simulink model "da2863_HW4_Simulink"  (R2023b)
settings: Solver=ode4  StartTime=0.0  StopTime=60  FixedStep=0.001  RelTol=1e-3
settings Model: Creator=Dhiya  LastModifiedBy=Dhiya

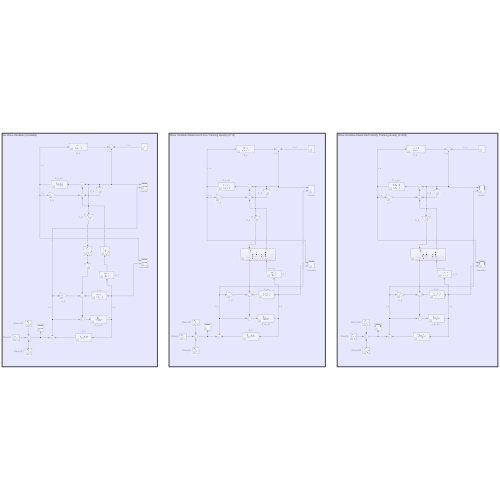
[thumbnail: Simulink's stored preview of the top-level diagram]
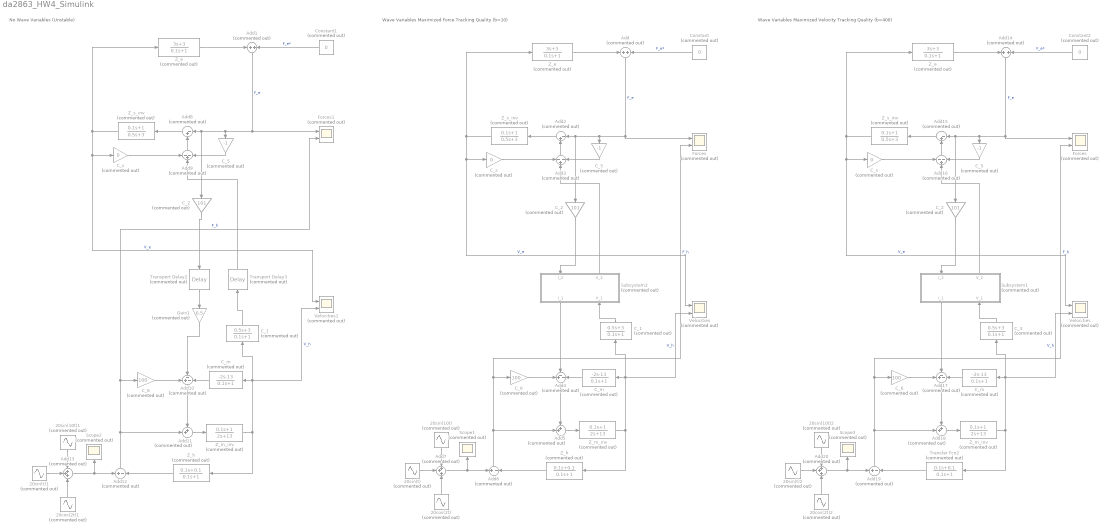
== system da2863_HW4_Simulink ==
  note: Wave Variables Maximized Velocity Tracking Quality (b=400)
  note: Wave Variables Maximized Force Tracking Quality (b=10)
  note: No Wave Variables (Unstable)
  20cos(2t) : Sin  Commented=on  Amplitude=20  Frequency=2  Phase=pi/2  SampleTime=0
  20cos(2t)1 : Sin  Commented=on  Amplitude=20  Frequency=2  Phase=pi/2  SampleTime=0
  20cos(2t)2 : Sin  Commented=on  Amplitude=20  Frequency=2  Phase=pi/2  SampleTime=0
  20sin(10t) : Sin  Commented=on  Amplitude=20  Frequency=10  SampleTime=0
  20sin(10t)1 : Sin  Commented=on  Amplitude=20  Frequency=10  SampleTime=0
  20sin(10t)2 : Sin  Commented=on  Amplitude=20  Frequency=10  SampleTime=0
  20sin(t) : Sin  Commented=on  Amplitude=20  SampleTime=0
  20sin(t)1 : Sin  Commented=on  Amplitude=20  SampleTime=0
  20sin(t)2 : Sin  Commented=on  Amplitude=20  SampleTime=0
  Add : Sum  Commented=on  Inputs=+|+
  Add1 : Sum  Commented=on  Inputs=+|+
  Add10 : Sum  Commented=on  Inputs=+--
  Add11 : Sum  Commented=on  Inputs=++|
  Add12 : Sum  Commented=on  Inputs=+|-
  Add13 : Sum  Commented=on  Inputs=+++
  Add14 : Sum  Commented=on  Inputs=+|+
  Add15 : Sum  Commented=on  Inputs=|-+
  Add16 : Sum  Commented=on  Inputs=-+-
  Add17 : Sum  Commented=on  Inputs=+--
  Add18 : Sum  Commented=on  Inputs=++|
  Add19 : Sum  Commented=on  Inputs=+|-
  Add2 : Sum  Commented=on  Inputs=|-+
  Add20 : Sum  Commented=on  Inputs=+++
  Add3 : Sum  Commented=on  Inputs=-+-
  Add4 : Sum  Commented=on  Inputs=+--
  Add5 : Sum  Commented=on  Inputs=++|
  Add6 : Sum  Commented=on  Inputs=+|-
  Add7 : Sum  Commented=on  Inputs=+++
  Add8 : Sum  Commented=on  Inputs=|-+
  Add9 : Sum  Commented=on  Inputs=-+-
  C_1 : TransferFcn  Commented=on  Numerator=[0.5 3]  Denominator=[0.1 1]
  "C_1 " : TransferFcn  Commented=on  Numerator=[0.5 3]  Denominator=[0.1 1]
  C_2 : Gain  Commented=on  Gain=101
  "C_2 " : Gain  Commented=on  Gain=101
  "C_2  " : Gain  Commented=on  Gain=101
  C_3 : TransferFcn  Commented=on  Numerator=[0.5 3]  Denominator=[0.1 1]
  C_5 : Gain  Commented=on  Gain=-1
  "C_5 " : Gain  Commented=on  Gain=-1
  "C_5  " : Gain  Commented=on  Gain=-1
  C_6 : Gain  Commented=on  Gain=100
  "C_6 " : Gain  Commented=on  Gain=100
  "C_6  " : Gain  Commented=on  Gain=100
  C_m : TransferFcn  Commented=on  Numerator=[-2 -13]  Denominator=[0.1 1]
  "C_m " : TransferFcn  Commented=on  Numerator=[-2 -13]  Denominator=[0.1 1]
  "C_m  " : TransferFcn  Commented=on  Numerator=[-2 -13]  Denominator=[0.1 1]
  C_s : Gain  Commented=on  Gain=0
  "C_s " : Gain  Commented=on  Gain=0
  "C_s  " : Gain  Commented=on  Gain=0
  Constant : Constant  Commented=on  Value=0
  Constant1 : Constant  Commented=on  Value=0
  Constant2 : Constant  Commented=on  Value=0
  Forces : Scope  Commented=on  NumInputPorts=2
  "Forces  " : Scope  Commented=on  NumInputPorts=2
  Forces1 : Scope  Commented=on  NumInputPorts=2
  Gain1 : Gain  Commented=on  Gain=0.5
  Scope1 : Scope  Commented=on
  Scope2 : Scope  Commented=on
  Scope3 : Scope  Commented=on
  Subsystem1 : Subsystem  Commented=on
      settings: PortSchema="{\"entries\":[{\"content\":{\"sides\":[{\"content\":{\"connectorIds\":[\"In1\",\"Out2\"]},\"type\":\"ConnectorPlacement.EquallySpacedRectSide\",\"uuid\":\"b47614d8-4282-40b8-98b5-b63f244bcd96\"},{\"content\":{\"connectorIds\":[\"Out1\",\"In2\"],\"side\":\"RIGHT\"},\"type\":\"ConnectorPlacement.EquallySpacedRectSide\",\"uuid\":\"bd48739f-0f37-4abb-b4a6-b3e75c0b7ee5\"},{\"content\":{\"side\":\"TOP\"},\"type\":\"ConnectorPlacement.EquallySpacedRectSide\",\"uuid\":\"b94baccd-0b63-48fd-a532-2b1ed6a2ffaa\"}]},\"type\":\"ConnectorPlacement.EquallySpacedConnector\",\"uuid\":\"3afc87c5-143e-47c9-ba54-3d5bde851d7b\"}],\"packageUris\":[\"http://schema.mathworks.com/mf0/Connector/R2020b\"],\"version\":\"1.0\"}"
  Subsystem2 : Subsystem  Commented=on
      settings: PortSchema="{\"entries\":[{\"content\":{\"sides\":[{\"content\":{\"connectorIds\":[\"In1\",\"Out2\"]},\"type\":\"ConnectorPlacement.EquallySpacedRectSide\",\"uuid\":\"b47614d8-4282-40b8-98b5-b63f244bcd96\"},{\"content\":{\"connectorIds\":[\"Out1\",\"In2\"],\"side\":\"RIGHT\"},\"type\":\"ConnectorPlacement.EquallySpacedRectSide\",\"uuid\":\"bd48739f-0f37-4abb-b4a6-b3e75c0b7ee5\"},{\"content\":{\"side\":\"TOP\"},\"type\":\"ConnectorPlacement.EquallySpacedRectSide\",\"uuid\":\"b94baccd-0b63-48fd-a532-2b1ed6a2ffaa\"}]},\"type\":\"ConnectorPlacement.EquallySpacedConnector\",\"uuid\":\"3afc87c5-143e-47c9-ba54-3d5bde851d7b\"}],\"packageUris\":[\"http://schema.mathworks.com/mf0/Connector/R2020b\"],\"version\":\"1.0\"}"
  Transfer Fcn2 : TransferFcn  Commented=on  Numerator=[0.1 0.1]  Denominator=[0.1 1]
  Transport Delay2 : TransportDelay  Commented=on  DelayTime=0.1
  Transport Delay3 : TransportDelay  Commented=on  DelayTime=0.1
  Velocities : Scope  Commented=on  NumInputPorts=2
  "Velocities  " : Scope  Commented=on  NumInputPorts=2
  Velocities1 : Scope  Commented=on  NumInputPorts=2
  Z_e : TransferFcn  Commented=on  Numerator=[3 3]  Denominator=[0.1 1]
  "Z_e " : TransferFcn  Commented=on  Numerator="[3  3]"  Denominator=[0.1 1]
  "Z_e  " : TransferFcn  Commented=on  Numerator=[3 3]  Denominator=[0.1 1]
  Z_h : TransferFcn  Commented=on  Numerator=[0.1 0.1]  Denominator=[0.1 1]
  "Z_h " : TransferFcn  Commented=on  Numerator=[0.1 0.1]  Denominator=[0.1 1]
  Z_m_inv : TransferFcn  Commented=on  Numerator=[0.1 1]  Denominator=[2 13]
  "Z_m_inv " : TransferFcn  Commented=on  Numerator=[0.1 1]  Denominator=[2 13]
  "Z_m_inv  " : TransferFcn  Commented=on  Numerator=[0.1 1]  Denominator=[2 13]
  Z_s_inv : TransferFcn  Commented=on  Numerator=[0.1 1]  Denominator=[0.5 3]
  "Z_s_inv " : TransferFcn  Commented=on  Numerator=[0.1 1]  Denominator=[0.5 3]
  "Z_s_inv  " : TransferFcn  Commented=on  Numerator=[0.1 1]  Denominator=[0.5 3]
  wires:
  Z_s_inv/1 -> Z_e/1, C_s/1, Velocities/1  "V_e"
  Add/1 -> C_2/1, Add2/1, C_5/1, Forces/1  "F_e"
  Add2/1 -> Z_s_inv/1
  C_s/1 -> Add3/1
  C_5/1 -> Add3/3
  Add3/1 -> Add2/2
  C_m/1 -> Add4/3
  Z_m_inv/1 -> "Z_h "/1, Velocities/2, C_m/1, C_1/1  "V_h"
  Add4/1 -> Add5/1
  Add5/1 -> Z_m_inv/1
  C_6/1 -> Add4/1
  Add6/1 -> Add5/2, Forces/2, C_6/1  "F_h"
  Add7/1 -> Scope1/1, Add6/1
  20sin(t)/1 -> Add7/2
  Constant/1 -> Add/2  "F_e*"
  C_1/1 -> Subsystem2/2(V_1)
  Z_e/1 -> Add/1
  "Z_h "/1 -> Add6/2
  C_2/1 -> Subsystem2/1(I_2)
  Subsystem2/1(I_1) -> Add4/2
  Gain1/1 -> Add10/2
  Constant1/1 -> Add1/2  "F_e*"
  Add8/1 -> "Z_s_inv "/1
  "C_2 "/1 -> Transport Delay2/1
  Transport Delay2/1 -> Gain1/1
  Z_h/1 -> Add12/2
  "C_6 "/1 -> Add10/1
  Transport Delay3/1 -> Add9/2
  Add13/1 -> Scope2/1, Add12/1
  "Z_m_inv "/1 -> Z_h/1, Velocities1/2, "C_m "/1, "C_1 "/1  "V_h"
  "Z_e "/1 -> Add1/1
  "C_m "/1 -> Add10/3
  Add11/1 -> "Z_m_inv "/1
  20sin(t)1/1 -> Add13/2
  20sin(10t)1/1 -> Add13/1
  Add9/1 -> Add8/2
  Add10/1 -> Add11/1
  "Z_s_inv "/1 -> "Z_e "/1, "C_s "/1, Velocities1/1  "V_e"
  20cos(2t)1/1 -> Add13/3
  "C_1 "/1 -> Transport Delay3/1
  Add12/1 -> Add11/2, Forces1/2, "C_6 "/1  "F_h"
  "C_s "/1 -> Add9/1
  "C_5 "/1 -> Add9/3
  Add1/1 -> "C_2 "/1, Add8/1, "C_5 "/1, Forces1/1  "F_e"
  Subsystem2/2(V_2) -> Add3/2
  20cos(2t)/1 -> Add7/3
  20sin(10t)/1 -> Add7/1
  20sin(10t)2/1 -> Add20/1
  20cos(2t)2/1 -> Add20/3
  Add15/1 -> "Z_s_inv  "/1
  "C_2  "/1 -> Subsystem1/1(I_2)
  Add17/1 -> Add18/1
  Transfer Fcn2/1 -> Add19/2
  20sin(t)2/1 -> Add20/2
  Constant2/1 -> Add14/2  "F_e*"
  "Z_m_inv  "/1 -> Transfer Fcn2/1, "Velocities  "/2, "C_m  "/1, C_3/1  "V_h"
  Add14/1 -> "C_2  "/1, Add15/1, "C_5  "/1, "Forces  "/1  "F_e"
  Add19/1 -> Add18/2, "Forces  "/2, "C_6  "/1  "F_h"
  Subsystem1/1(I_1) -> Add17/2
  "C_m  "/1 -> Add17/3
  Add18/1 -> "Z_m_inv  "/1
  "C_6  "/1 -> Add17/1
  "Z_e  "/1 -> Add14/1
  "C_5  "/1 -> Add16/3
  Add20/1 -> Scope3/1, Add19/1
  "C_s  "/1 -> Add16/1
  "Z_s_inv  "/1 -> "Z_e  "/1, "C_s  "/1, "Velocities  "/1  "V_e"
  Subsystem1/2(V_2) -> Add16/2
  Add16/1 -> Add15/2
  C_3/1 -> Subsystem1/2(V_1)

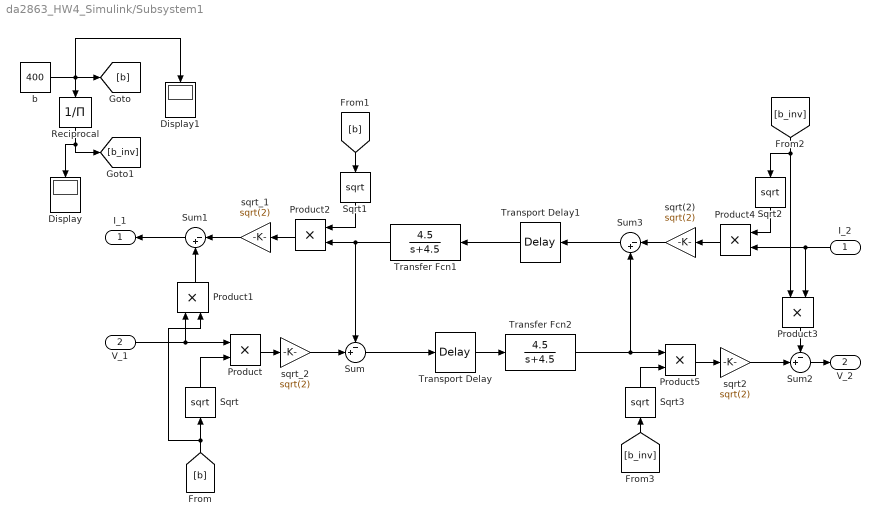
== system da2863_HW4_Simulink/Subsystem1 ==
  I_2 : Inport
  V_1 : Inport  Port=2
  Display : Display
  Display1 : Display
      settings: Decimation=100
  Product{,1..5} (6 alike) : Product
  Reciprocal : Product  Inputs=/
  Sqrt{,1..3} (4 alike) : Sqrt
  Sum : Sum  Inputs=-+|
  Sum1 : Sum  Inputs=|-+
  Sum2 : Sum  Inputs=-+|
  Sum3 : Sum  Inputs=|-+
  Transfer Fcn1 : TransferFcn  Numerator=[4.5]  Denominator=[1 4.5]
  Transfer Fcn2 : TransferFcn  Numerator=[4.5]  Denominator=[1 4.5]
  Transport Delay : TransportDelay  DelayTime=0.1
  Transport Delay1 : TransportDelay  DelayTime=0.1
  b : Constant  Value=400
  sqrt(2) : Gain  Gain=sqrt(2)
  sqrt2 : Gain  Gain=sqrt(2)
  sqrt_1 : Gain  Gain=sqrt(2)
  sqrt_2 : Gain  Gain=sqrt(2)
  I_1 : Outport
  V_2 : Outport  Port=2
  wires:
  V_1/1 -> Product1/1, Product/1
  Product/1 -> sqrt_2/1
  sqrt_2/1 -> Sum/2
  Sqrt/1 -> Product/2
  Product1/1 -> Sum1/2
  sqrt_1/1 -> Sum1/1
  Product2/1 -> sqrt_1/1
  Transport Delay1/1 -> Transfer Fcn1/1
  b/1 -> Display1/1, [b], Reciprocal/1
  [b] -> Product1/2, Sqrt/1
  [b] -> Sqrt1/1
  Sqrt1/1 -> Product2/1
  Sum1/1 -> I_1/1
  Reciprocal/1 -> Display/1, [b_inv]
  I_2/1 -> Product3/2, Product4/2
  [b_inv] -> Sqrt2/1, Product3/1
  Product3/1 -> Sum2/1
  Sum2/1 -> V_2/1
  Sqrt2/1 -> Product4/1
  Product4/1 -> sqrt(2)/1
  sqrt(2)/1 -> Sum3/1
  Transport Delay/1 -> Transfer Fcn2/1
  Product5/1 -> sqrt2/1
  [b_inv] -> Sqrt3/1
  Sqrt3/1 -> Product5/2
  sqrt2/1 -> Sum2/2
  Sum3/1 -> Transport Delay1/1
  Sum/1 -> Transport Delay/1
  Transfer Fcn1/1 -> Sum/1, Product2/2
  Transfer Fcn2/1 -> Product5/1, Sum3/2

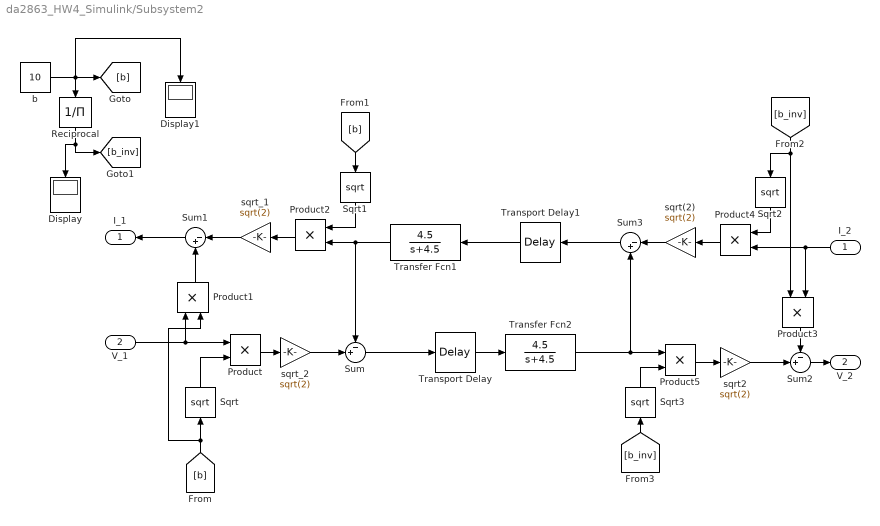
== system da2863_HW4_Simulink/Subsystem2 ==
  I_2 : Inport
  V_1 : Inport  Port=2
  Display : Display
  Display1 : Display
      settings: Decimation=100
  Product{,1..5} (6 alike) : Product
  Reciprocal : Product  Inputs=/
  Sqrt{,1..3} (4 alike) : Sqrt
  Sum : Sum  Inputs=-+|
  Sum1 : Sum  Inputs=|-+
  Sum2 : Sum  Inputs=-+|
  Sum3 : Sum  Inputs=|-+
  Transfer Fcn1 : TransferFcn  Numerator=[4.5]  Denominator=[1 4.5]
  Transfer Fcn2 : TransferFcn  Numerator=[4.5]  Denominator=[1 4.5]
  Transport Delay : TransportDelay  DelayTime=0.1
  Transport Delay1 : TransportDelay  DelayTime=0.1
  b : Constant  Value=10
  sqrt(2) : Gain  Gain=sqrt(2)
  sqrt2 : Gain  Gain=sqrt(2)
  sqrt_1 : Gain  Gain=sqrt(2)
  sqrt_2 : Gain  Gain=sqrt(2)
  I_1 : Outport
  V_2 : Outport  Port=2
  wires:
  V_1/1 -> Product1/1, Product/1
  Product/1 -> sqrt_2/1
  sqrt_2/1 -> Sum/2
  Sqrt/1 -> Product/2
  Product1/1 -> Sum1/2
  sqrt_1/1 -> Sum1/1
  Product2/1 -> sqrt_1/1
  Transport Delay1/1 -> Transfer Fcn1/1
  b/1 -> Display1/1, [b], Reciprocal/1
  [b] -> Product1/2, Sqrt/1
  [b] -> Sqrt1/1
  Sqrt1/1 -> Product2/1
  Sum1/1 -> I_1/1
  Reciprocal/1 -> Display/1, [b_inv]
  I_2/1 -> Product3/2, Product4/2
  [b_inv] -> Sqrt2/1, Product3/1
  Product3/1 -> Sum2/1
  Sum2/1 -> V_2/1
  Sqrt2/1 -> Product4/1
  Product4/1 -> sqrt(2)/1
  sqrt(2)/1 -> Sum3/1
  Transport Delay/1 -> Transfer Fcn2/1
  Product5/1 -> sqrt2/1
  [b_inv] -> Sqrt3/1
  Sqrt3/1 -> Product5/2
  sqrt2/1 -> Sum2/2
  Sum3/1 -> Transport Delay1/1
  Sum/1 -> Transport Delay/1
  Transfer Fcn1/1 -> Sum/1, Product2/2
  Transfer Fcn2/1 -> Product5/1, Sum3/2
